simulink model "MMNQueue"  (R2016b)
settings: Solver=VariableStepAuto  StartTime=0.0  StopTime=40000  RelTol=1e-6  EnableMultiTasking=on
values from neighbouring files (symbols this model uses):
  lambda = x(i) * N    [sim_mmn_queue.m]
  n = x    [model_mmn_queue.m]
undefined symbols (not defined in the file or in its folder): m
libraries: simulink x1, dspstat3 x1
settings Model: Creator=The MathWorks, Inc.  LastModifiedBy=baites
settings DataIOCC: LimitDataPoints=on  SaveFormat=Array
settings OptimizationCC: LifeSpan=inf
settings DebuggingCC: AllowSymbolicDim=off  SFUnexpectedBacktrackingDiag=warning  SFNoUnconditionalDefaultTransitionDiag=warning  SFExecutionAtInitializationDiag=none
settings ModelReferenceCC: PropagateSignalLabelsOutOfModel=off
settings GRTTargetCC: TargetLangStandard=C89/C90 (ANSI)  GeneratePreprocessorConditionals=Disable all
settings ConfigComp: CovMetricSettings=dw  CovHtmlReporting=on  CovSaveCumulativeToWorkspaceVar=on  CovSaveSingleToWorkspaceVar=on  CovExternalEMLEnable=off  CovSFcnEnable=off

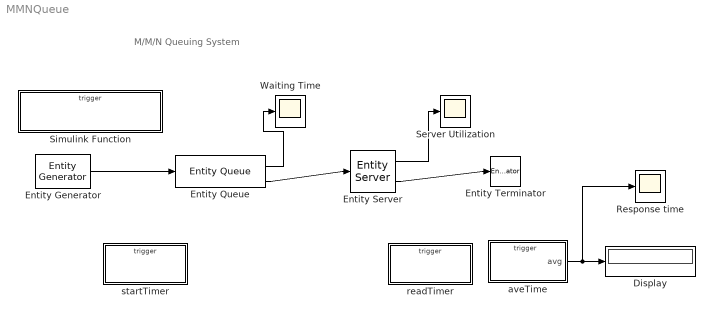
== system MMNQueue ==
  note: M/M/N Queuing System
  Display : Display
  Entity Generator : EntityGenerator  OutputPortMessageModes=m  TimeSource=MATLAB action  IntergenerationTimeAction=dt = exponentialArrivalTime();  AttributeName=Attribute1|Timer  AttributeInitialValue=1|0  EntityType=Structured  EntityTypeName=Entity
  Entity Queue : EntityQueue  InputPortMessageModes=m  OutputPortMessageModes=n,m  Capacity=Inf  EntryAction=entity.Timer = startTimer();  AverageWait=on
      settings: OutputPortMap=o2,o5
  Entity Server : EntityServer  InputPortMessageModes=m  OutputPortMessageModes=n,m  Capacity=N  ServiceTimeSource=MATLAB action  ServiceTimeAction=|  ExitAction=|  Utilization=on
      ServiceTimeAction=|
      | % Exponential service time with rate 1
      | dt   = -1/mu * log(1 - rand());
      ExitAction=|
      | delta = readTimer(entity.Timer);
      | aveTime(delta);
      settings: OutputPortMap=o5,o9
  Entity Terminator : EntityTerminator  InputPortMessageModes=m
  Response time : Scope
  Server Utilization : Scope
  Simulink Function : Subsystem  TreatAsAtomicUnit=on
  Waiting Time : Scope
  aveTime : Subsystem  TreatAsAtomicUnit=on
  readTimer : Subsystem  TreatAsAtomicUnit=on
  "startTimer " : Subsystem  TreatAsAtomicUnit=on
  wires:
  Entity Generator/1 -> Entity Queue/1
  Entity Queue/2 -> Entity Server/1
  Entity Server/2 -> Entity Terminator/1
  Entity Queue/1 -> Waiting Time/1
  Entity Server/1 -> Server Utilization/1
  aveTime/1(avg) -> Response time/1, Display/1

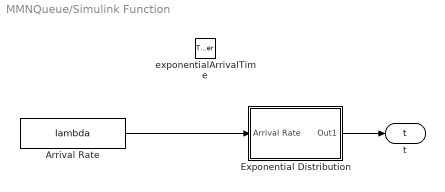
== system MMNQueue/Simulink Function ==
  exponentialArrivalTime : TriggerPort  TriggerType=function-call  IsSimulinkFunction=on  FunctionName=exponentialArrivalTime  VariantControl=Variant
  Arrival Rate : Constant  Value=lambda  SampleTime=-1
  Exponential Distribution : Subsystem
  t : ArgOut  DisableCoverage=on  ArgumentName=t
  wires:
  Arrival Rate/1 -> Exponential Distribution/1(Arrival Rate)
  Exponential Distribution/1(Out1) -> t/1

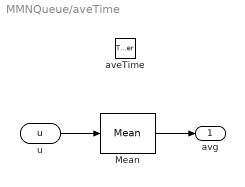
== system MMNQueue/aveTime ==
  aveTime : TriggerPort  TriggerType=function-call  IsSimulinkFunction=on  FunctionName=aveTime  VariantControl=Variant
  Mean : dspstat3/Mean  run=on  reset_popup=None  directionMode=Each column  dimension=1  roiEnable=off  roiType=Rectangles  roiPortion=Entire ROI  roiOutput=Individual statistics for each ROI  roiFlag=off  outputDataTypeStr=Inherit: Same as accumulator  outputLastDataTypeStr=Inherit: Same as accumulator  outputMin=[]  outputMax=[]  roundingMode=Floor  overflowMode=off
  u : ArgIn  DisableCoverage=on  ArgumentName=u
  avg : Outport
  wires:
  u/1 -> Mean/1
  Mean/1 -> avg/1

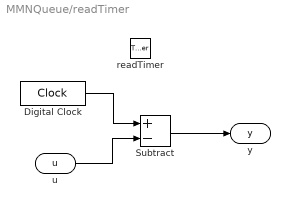
== system MMNQueue/readTimer ==
  readTimer : TriggerPort  TriggerType=function-call  IsSimulinkFunction=on  FunctionName=readTimer  VariantControl=Variant
  Digital Clock : DigitalClock  SampleTime=-1
  Subtract : Sum  Inputs=+-
  u : ArgIn  DisableCoverage=on  ArgumentName=u
  y : ArgOut  DisableCoverage=on  ArgumentName=y
  wires:
  u/1 -> Subtract/2
  Subtract/1 -> y/1
  Digital Clock/1 -> Subtract/1

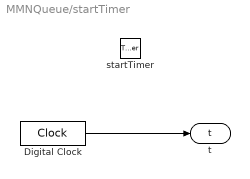
== system MMNQueue/startTimer  ==
  startTimer : TriggerPort  TriggerType=function-call  IsSimulinkFunction=on  FunctionName=startTimer  VariantControl=Variant
  Digital Clock : DigitalClock  SampleTime=-1
  t : ArgOut  DisableCoverage=on  ArgumentName=t
  wires:
  Digital Clock/1 -> t/1

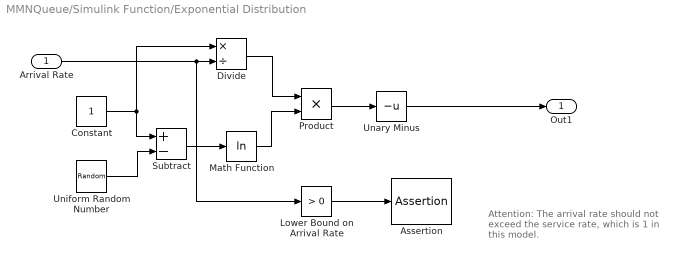
== system MMNQueue/Simulink Function/Exponential Distribution ==
  note: Attention: The arrival rate
      | should not exceed the service
      | rate, which is 1 in this model.
  Arrival Rate : Inport
  Assertion : Assertion
  Constant : Constant
  Divide : Product  Inputs=*/
  Lower Bound on Arrival Rate : simulink/Logic and Bit Operations/Compare To Constant  relop=>  const=0  OutDataTypeStr=uint8  ZeroCross=off
  Math Function : Math  Operator=log  SaturateOnIntegerOverflow=on
  Product : Product  RndMeth=Zero
  Subtract : Sum  Inputs=+-
  Unary Minus : UnaryMinus
  Uniform Random Number : UniformRandomNumber  Minimum=0  Seed=12345
  Out1 : Outport
  wires:
  Arrival Rate/1 -> Divide/2, Lower Bound on Arrival Rate/1
  Unary Minus/1 -> Out1/1
  Product/1 -> Unary Minus/1
  Math Function/1 -> Product/2
  Divide/1 -> Product/1
  Constant/1 -> Divide/1, Subtract/1
  Uniform Random Number/1 -> Subtract/2
  Lower Bound on Arrival Rate/1 -> Assertion/1
  Subtract/1 -> Math Function/1
